simulink library "lib_component"  (Simulink 7.7)
settings: Solver=ode45  StartTime=0.0  StopTime=10.0  RelTol=1e-3
undefined symbols (not defined in the file): Earth, four_skew_D0, four_skew_D1, four_skew_D2, four_skew_D3, four_skew_D4, GAS_k, GAS_seed1, GAS_tau, GAS_Vnoise, GAS_Vref, GPS_position_noise, GPS_position_seed, GPS_time_noise, GPS_time_seed, GYRO_bx, GYRO_by, GYRO_bz, GYRO_nu, GYRO_nv, GYRO_omega, GYRO_seed1, GYRO_seed2, GYRO_zeta, MTQ_k, MTQ_tau, noise_sampling_rate, NSAS_ang_limit, NSAS_seed1, NSAS_seed2, NSAS_x_noise, NSAS_y_noise, RW_Gamp, RW_J, RW_kE, RW_kL, RW_kT, RW_LM, RW_RM, RW_Rsc, RW_T1, RW_T2, STT_AD_prob, STT_FOV, STT_moon_ang_limit, STT_sun_ang_limit, STT_x_noise, STT_y_noise, STT_z_noise, three_one_skew_D0, three_one_skew_D1, three_one_skew_D2, three_one_skew_D3, three_one_skew_D4, three_one_skew_matrix, WGS84
libraries: lib_component x11, simulink x5, aerolibutil x4, lib_util x2, lib_env x2, aerolibtransform2 x1, vrlib x1
settings Model: Creator=kkamiya  LastModifiedBy=yamaurashusaku

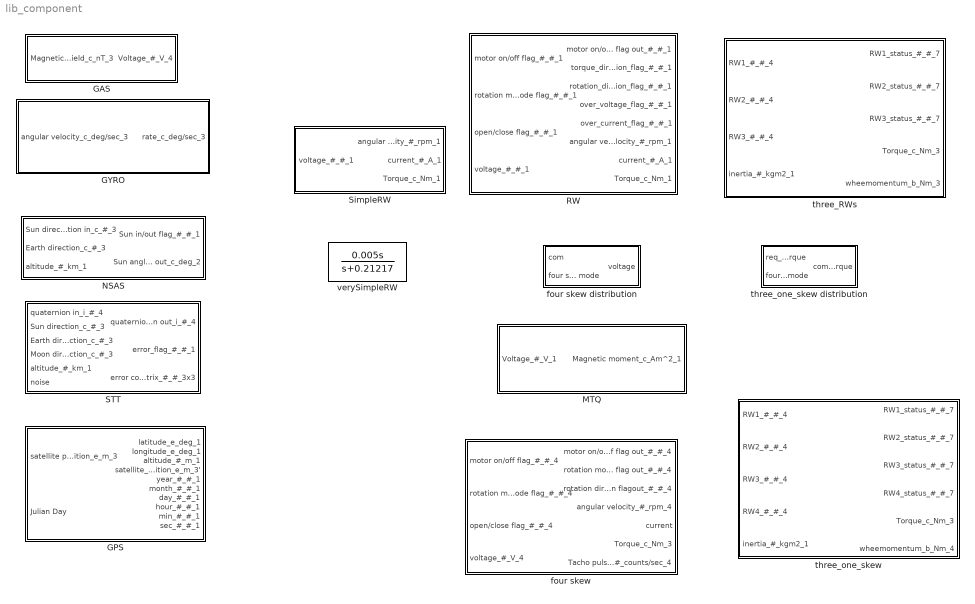
== system lib_component ==
  GAS : Subsystem
  GPS : Subsystem
  GYRO : Subsystem
  MTQ : Subsystem
  NSAS : Subsystem
  RW : Subsystem
  STT : Subsystem
  SimpleRW : Subsystem
  four skew : Subsystem
  four skew distribution : Subsystem
  three_RWs : Subsystem  AncestorBlock=lib_component/three_one_skew
  three_one_skew : Subsystem
  three_one_skew distribution : Subsystem
  verySimpleRW : TransferFcn  Numerator=[0.005 0]  Denominator=[1 0.21217]

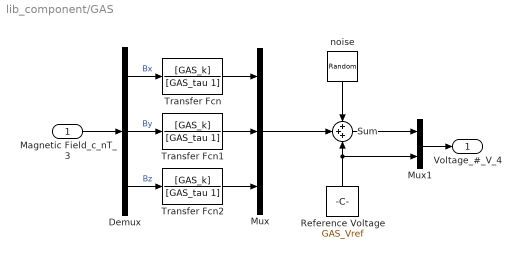
== system lib_component/GAS ==
  Magnetic Field_c_nT_3 : Inport
  Demux : Demux  Outputs=3
  Mux : Mux  Inputs=3
  Mux1 : Mux  Inputs=2
  Reference Voltage : Constant  Value=GAS_Vref
  Sum : Sum  Inputs=+++
  Transfer Fcn : TransferFcn  Numerator=[GAS_k]  Denominator=[GAS_tau 1]
  Transfer Fcn1 : TransferFcn  Numerator=[GAS_k]  Denominator=[GAS_tau 1]
  Transfer Fcn2 : TransferFcn  Numerator=[GAS_k]  Denominator=[GAS_tau 1]
  noise : RandomNumber  Mean=[0 0 0]  Variance=[GAS_Vnoise*GAS_Vnoise GAS_Vnoise*GAS_Vnoise GAS_Vnoise*GAS_Vnoise]  Seed=GAS_seed1  SampleTime=noise_sampling_rate
  Voltage_#_V_4 : Outport
  wires:
  Demux/2 -> Transfer Fcn1/1  "By"
  Demux/3 -> Transfer Fcn2/1  "Bz"
  Demux/1 -> Transfer Fcn/1  "Bx"
  Transfer Fcn2/1 -> Mux/3
  Transfer Fcn1/1 -> Mux/2
  Transfer Fcn/1 -> Mux/1
  Mux/1 -> Sum/2
  Mux1/1 -> Voltage_#_V_4/1
  Reference Voltage/1 -> Sum/3, Mux1/2
  Sum/1 -> Mux1/1
  Magnetic Field_c_nT_3/1 -> Demux/1
  noise/1 -> Sum/1

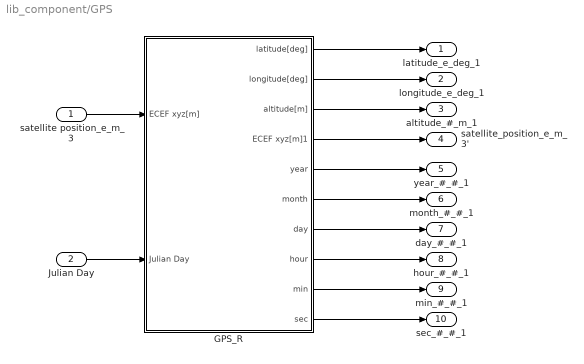
== system lib_component/GPS ==
  satellite position_e_m_3 : Inport
  Julian Day : Inport  Port=2
  GPS_R : Subsystem
  latitude_e_deg_1 : Outport
  longitude_e_deg_1 : Outport  Port=2
  altitude_#_m_1 : Outport  Port=3
  satellite_position_e_m_3' : Outport  Port=4
  year_#_#_1 : Outport  Port=5
  month_#_#_1 : Outport  Port=6
  day_#_#_1 : Outport  Port=7
  hour_#_#_1 : Outport  Port=8
  min_#_#_1 : Outport  Port=9
  sec_#_#_1 : Outport  Port=10
  wires:
  Julian Day/1 -> GPS_R/2(Julian Day)
  satellite position_e_m_3/1 -> GPS_R/1(ECEF xyz[m])
  GPS_R/1(latitude[deg]) -> latitude_e_deg_1/1
  GPS_R/2(longitude[deg]) -> longitude_e_deg_1/1
  GPS_R/3(altitude[m]) -> altitude_#_m_1/1
  GPS_R/4(ECEF xyz[m]1) -> satellite_position_e_m_3'/1
  GPS_R/5(year) -> year_#_#_1/1
  GPS_R/6(month) -> month_#_#_1/1
  GPS_R/7(day) -> day_#_#_1/1
  GPS_R/8(hour) -> hour_#_#_1/1
  GPS_R/9(min) -> min_#_#_1/1
  GPS_R/10(sec) -> sec_#_#_1/1

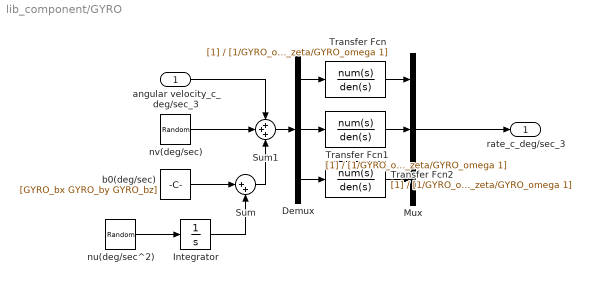
== system lib_component/GYRO ==
  angular velocity_c_deg/sec_3 : Inport
  Demux : Demux  Outputs=3
  Integrator : Integrator
  Mux : Mux  Inputs=3
  Sum : Sum  Inputs=|++
  Sum1 : Sum  Inputs=+++
  Transfer Fcn : TransferFcn  Denominator=[1/GYRO_omega/GYRO_omega 2*GYRO_zeta/GYRO_omega 1]
  Transfer Fcn1 : TransferFcn  Denominator=[1/GYRO_omega/GYRO_omega 2*GYRO_zeta/GYRO_omega 1]
  Transfer Fcn2 : TransferFcn  Denominator=[1/GYRO_omega/GYRO_omega 2*GYRO_zeta/GYRO_omega 1]
  b0(deg/sec) : Constant  Value=[GYRO_bx GYRO_by GYRO_bz]
  nu(deg/sec^2) : RandomNumber  Mean=[0 0 0]  Variance=[GYRO_nu*GYRO_nu GYRO_nu*GYRO_nu GYRO_nu*GYRO_nu]  Seed=GYRO_seed2  SampleTime=noise_sampling_rate
  nv(deg/sec) : RandomNumber  Mean=[0 0 0]  Variance=[GYRO_nv*GYRO_nv GYRO_nv*GYRO_nv GYRO_nv*GYRO_nv]  Seed=GYRO_seed1  SampleTime=noise_sampling_rate
  rate_c_deg/sec_3 : Outport
  wires:
  Transfer Fcn/1 -> Mux/1
  Transfer Fcn1/1 -> Mux/2
  Transfer Fcn2/1 -> Mux/3
  nu(deg/sec^2)/1 -> Integrator/1
  b0(deg/sec)/1 -> Sum/1
  nv(deg/sec)/1 -> Sum1/2
  Sum/1 -> Sum1/3
  angular velocity_c_deg/sec_3/1 -> Sum1/1
  Sum1/1 -> Demux/1
  Demux/2 -> Transfer Fcn1/1
  Demux/1 -> Transfer Fcn/1
  Demux/3 -> Transfer Fcn2/1
  Mux/1 -> rate_c_deg/sec_3/1
  Integrator/1 -> Sum/2

== system lib_component/MTQ ==
  Voltage_#_V_1 : Inport
  Transfer Fcn : TransferFcn  Numerator=[MTQ_k]  Denominator=[MTQ_tau 1]
  Magnetic moment_c_Am^2_1 : Outport
  wires:
  Voltage_#_V_1/1 -> Transfer Fcn/1
  Transfer Fcn/1 -> Magnetic moment_c_Am^2_1/1

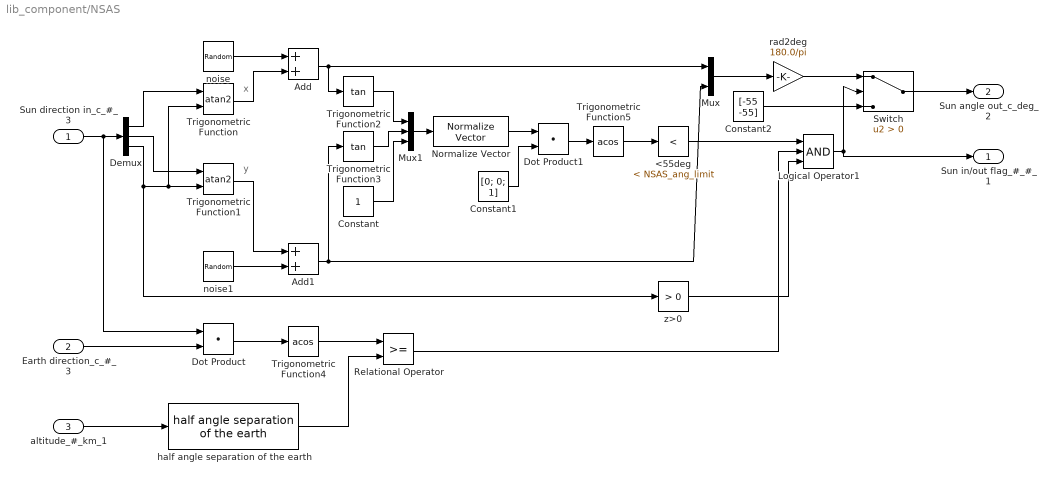
== system lib_component/NSAS ==
  note: x
  note: y
  Sun direction in_c_#_3 : Inport
  Earth direction_c_#_3 : Inport  Port=2
  altitude_#_km_1 : Inport  Port=3
  <55deg : simulink/Logic and Bit Operations/Compare To Constant  SystemSampleTime=-1  relop=<  const=NSAS_ang_limit  LogicOutDataTypeMode=uint8
  Add : Sum
  Add1 : Sum
  Constant : Constant
  Constant1 : Constant  Value=[0; 0; 1]
  Constant2 : Constant  Value=[-55 -55]
  Demux : Demux  Outputs=3
  Dot Product : DotProduct  InputSameDT=on  OutDataTypeStr=Inherit: Inherit via internal rule
  Dot Product1 : DotProduct  InputSameDT=on  OutDataTypeStr=Inherit: Inherit via internal rule
  Logical Operator1 : Logic  Inputs=3  AllPortsSameDT=off  OutDataTypeStr=boolean
  Mux : Mux  Inputs=2
  Mux1 : Mux  Inputs=3
  Normalize Vector : vrlib/Utilities/Normalize Vector  SystemSampleTime=-1  maxzero=0
  Relational Operator : RelationalOperator  OutDataTypeStr=boolean
  Switch : Switch  Criteria=u2 > Threshold
  Trigonometric Function : Trigonometry  Operator=atan2
  Trigonometric Function1 : Trigonometry  Operator=atan2
  Trigonometric Function2 : Trigonometry  Operator=tan
  Trigonometric Function3 : Trigonometry  Operator=tan
  Trigonometric Function4 : Trigonometry  Operator=acos
  Trigonometric Function5 : Trigonometry  Operator=acos
  half angle separation of the earth : lib_env/half angle separation of the earth  SystemSampleTime=-1
  noise : RandomNumber  Variance=NSAS_x_noise*NSAS_x_noise  Seed=NSAS_seed1  SampleTime=noise_sampling_rate
  noise1 : RandomNumber  Variance=NSAS_y_noise*NSAS_y_noise  Seed=NSAS_seed2  SampleTime=noise_sampling_rate
  rad2deg : Gain  Gain=180.0/pi
  z>0 : simulink/Logic and Bit Operations/Compare To Constant  SystemSampleTime=-1  relop=>  const=0  LogicOutDataTypeMode=uint8
  Sun in/out flag_#_#_1 : Outport
  Sun angle out_c_deg_2 : Outport  Port=2
  wires:
  noise1/1 -> Add1/2
  noise/1 -> Add/1
  Add/1 -> Mux/1, Trigonometric Function2/1
  Mux/1 -> rad2deg/1
  Switch/1 -> Sun angle out_c_deg_2/1
  Constant2/1 -> Switch/3
  Sun direction in_c_#_3/1 -> Demux/1, Dot Product/1
  Demux/2 -> Trigonometric Function1/1
  Demux/3 -> Trigonometric Function/2, Trigonometric Function1/2, z>0/1
  Demux/1 -> Trigonometric Function/1
  Trigonometric Function1/1 -> Add1/1
  Trigonometric Function/1 -> Add/2
  altitude_#_km_1/1 -> half angle separation of the earth/1
  Earth direction_c_#_3/1 -> Dot Product/2
  Dot Product/1 -> Trigonometric Function4/1
  half angle separation of the earth/1 -> Relational Operator/2
  Trigonometric Function4/1 -> Relational Operator/1
  Relational Operator/1 -> Logical Operator1/2
  Logical Operator1/1 -> Sun in/out flag_#_#_1/1, Switch/2
  Add1/1 -> Mux/2, Trigonometric Function3/1
  rad2deg/1 -> Switch/1
  <55deg/1 -> Logical Operator1/1
  Trigonometric Function2/1 -> Mux1/1
  Trigonometric Function3/1 -> Mux1/2
  Constant/1 -> Mux1/3
  Mux1/1 -> Normalize Vector/1
  Normalize Vector/1 -> Dot Product1/1
  Constant1/1 -> Dot Product1/2
  Dot Product1/1 -> Trigonometric Function5/1
  Trigonometric Function5/1 -> <55deg/1
  z>0/1 -> Logical Operator1/3

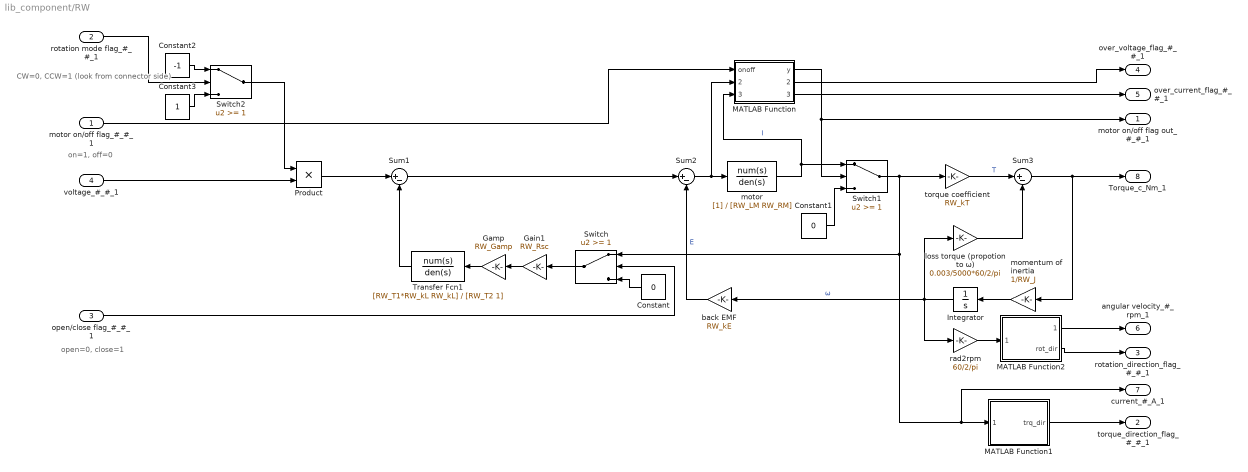
== system lib_component/RW ==
  note: CW=0, CCW=1
      | (look from connector side)
  note: open=0, close=1
  note: on=1, off=0
  motor on/off flag_#_#_1 : Inport
  rotation mode flag_#_#_1 : Inport  Port=2
  open/close flag_#_#_1 : Inport  Port=3
  voltage_#_#_1 : Inport  Port=4
  Constant : Constant  Value=0
  Constant1 : Constant  Value=0
  Constant2 : Constant  Value=-1
  Constant3 : Constant
  Gain1 : Gain  Gain=RW_Rsc
  Gamp : Gain  Gain=RW_Gamp
  Integrator : Integrator
  MATLAB Function : Stateflow chart  TreatAsAtomicUnit=on
  MATLAB Function1 : Stateflow chart  TreatAsAtomicUnit=on
  MATLAB Function2 : Stateflow chart  TreatAsAtomicUnit=on
  Product : Product  RndMeth=Zero
  Sum1 : Sum  Inputs=|+-
  Sum2 : Sum  Inputs=|+-
  Sum3 : Sum  Inputs=|+-
  Switch : Switch  Threshold=1
  Switch1 : Switch  Threshold=1
  Switch2 : Switch  Threshold=1
  Transfer Fcn1 : TransferFcn  Numerator=[RW_T1*RW_kL RW_kL]  Denominator=[RW_T2 1]
  back EMF : Gain  Gain=RW_kE
  loss torque (propotion to ω) : Gain  Gain=0.003/5000*60/2/pi
  momentum of inertia : Gain  Gain=1/RW_J
  motor : TransferFcn  Denominator=[RW_LM RW_RM]
  rad2rpm : Gain  Gain=60/2/pi
  torque coefficient : Gain  Gain=RW_kT
  motor on/off flag out_#_#_1 : Outport
  torque_direction_flag_#_#_1 : Outport  Port=2
  rotation_direction_flag_#_#_1 : Outport  Port=3
  over_voltage_flag_#_#_1 : Outport  Port=4
  over_current_flag_#_#_1 : Outport  Port=5
  angular velocity_#_rpm_1 : Outport  Port=6
  current_#_A_1 : Outport  Port=7
  Torque_c_Nm_1 : Outport  Port=8
  wires:
  Integrator/1 -> loss torque (propotion to ω)/1, back EMF/1, rad2rpm/1  "ω"
  momentum of inertia/1 -> Integrator/1
  torque coefficient/1 -> Sum3/1  "T"
  Sum2/1 -> motor/1, MATLAB Function/2(voltage)
  Gamp/1 -> Transfer Fcn1/1
  Gain1/1 -> Gamp/1
  rotation mode flag_#_#_1/1 -> Switch2/2
  open/close flag_#_#_1/1 -> Switch/2
  Constant/1 -> Switch/3
  Transfer Fcn1/1 -> Sum1/2
  Switch/1 -> Gain1/1
  rad2rpm/1 -> MATLAB Function2/1(omega)
  back EMF/1 -> Sum2/2  "E"
  Sum3/1 -> momentum of inertia/1, Torque_c_Nm_1/1
  loss torque (propotion to ω)/1 -> Sum3/2
  Constant2/1 -> Switch2/1
  Constant3/1 -> Switch2/3
  voltage_#_#_1/1 -> Product/2
  Switch2/1 -> Product/1
  Product/1 -> Sum1/1
  Switch1/1 -> torque coefficient/1, Switch/1, MATLAB Function1/1(current), current_#_A_1/1
  motor on/off flag_#_#_1/1 -> MATLAB Function/1(onoff)
  motor/1 -> Switch1/1, MATLAB Function/3(current)  "I"
  Constant1/1 -> Switch1/3
  MATLAB Function/1(y) -> Switch1/2, motor on/off flag out_#_#_1/1
  Sum1/1 -> Sum2/1
  MATLAB Function1/1(trq_dir) -> torque_direction_flag_#_#_1/1
  MATLAB Function2/2(rot_dir) -> rotation_direction_flag_#_#_1/1
  MATLAB Function2/1(omega_out) -> angular velocity_#_rpm_1/1
  MATLAB Function/2(over_voltage) -> over_voltage_flag_#_#_1/1
  MATLAB Function/3(over_current) -> over_current_flag_#_#_1/1

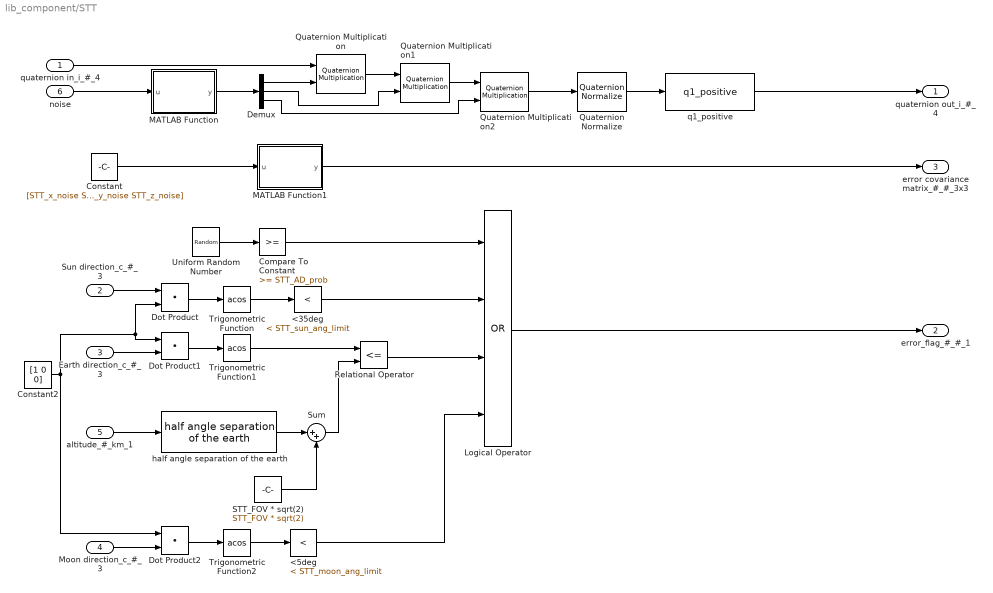
== system lib_component/STT ==
  quaternion in_i_#_4 : Inport
  Sun direction_c_#_3 : Inport  Port=2
  Earth direction_c_#_3 : Inport  Port=3
  Moon direction_c_#_3 : Inport  Port=4
  altitude_#_km_1 : Inport  Port=5
  noise : Inport  Port=6
  <35deg : simulink/Logic and Bit Operations/Compare To Constant  SystemSampleTime=-1  relop=<  const=STT_sun_ang_limit  LogicOutDataTypeMode=uint8
  <5deg : simulink/Logic and Bit Operations/Compare To Constant  SystemSampleTime=-1  relop=<  const=STT_moon_ang_limit  LogicOutDataTypeMode=uint8
  Compare To Constant : simulink/Logic and Bit Operations/Compare To Constant  SystemSampleTime=-1  relop=>=  const=STT_AD_prob  LogicOutDataTypeMode=uint8
  Constant : Constant  Value=[STT_x_noise STT_y_noise STT_z_noise]  SampleTime=0
  Constant2 : Constant  Value=[1 0 0]
  Demux : Demux  Outputs=3
  Dot Product : DotProduct  InputSameDT=on  OutDataTypeStr=Inherit: Inherit via internal rule
  Dot Product1 : DotProduct  InputSameDT=on  OutDataTypeStr=Inherit: Inherit via internal rule
  Dot Product2 : DotProduct  InputSameDT=on  OutDataTypeStr=Inherit: Inherit via internal rule
  Logical Operator : Logic  Operator=OR  Inputs=4  AllPortsSameDT=off  OutDataTypeStr=boolean
  MATLAB Function : Stateflow chart  TreatAsAtomicUnit=on
  MATLAB Function1 : Stateflow chart  TreatAsAtomicUnit=on
  Quaternion Multiplication : aerolibutil/Quaternion Multiplication  SystemSampleTime=-1
  Quaternion Multiplication1 : aerolibutil/Quaternion Multiplication  SystemSampleTime=-1
  Quaternion Multiplication2 : aerolibutil/Quaternion Multiplication  SystemSampleTime=-1
  Quaternion Normalize : aerolibutil/Quaternion Normalize  SystemSampleTime=-1
  Relational Operator : RelationalOperator  Operator=<=  OutDataTypeStr=boolean
  STT_FOV * sqrt(2) : Constant  Value=STT_FOV * sqrt(2)
  Sum : Sum  Inputs=|++
  Trigonometric Function : Trigonometry  Operator=acos
  Trigonometric Function1 : Trigonometry  Operator=acos
  Trigonometric Function2 : Trigonometry  Operator=acos
  Uniform Random Number : UniformRandomNumber  Minimum=0  SampleTime=noise_sampling_rate
  half angle separation of the earth : lib_env/half angle separation of the earth  SystemSampleTime=-1
  q1_positive : lib_util/q1_positive  SystemSampleTime=-1
  quaternion out_i_#_4 : Outport
  error_flag_#_#_1 : Outport  Port=2
  error covariance matrix_#_#_3x3 : Outport  Port=3
  wires:
  Dot Product2/1 -> Trigonometric Function2/1
  <5deg/1 -> Logical Operator/4
  Trigonometric Function2/1 -> <5deg/1
  Moon direction_c_#_3/1 -> Dot Product2/2
  <35deg/1 -> Logical Operator/2
  Trigonometric Function/1 -> <35deg/1
  Dot Product1/1 -> Trigonometric Function1/1
  Dot Product/1 -> Trigonometric Function/1
  Constant2/1 -> Dot Product2/1, Dot Product1/1, Dot Product/2
  Logical Operator/1 -> error_flag_#_#_1/1
  Compare To Constant/1 -> Logical Operator/1
  Earth direction_c_#_3/1 -> Dot Product1/2
  Sun direction_c_#_3/1 -> Dot Product/1
  Uniform Random Number/1 -> Compare To Constant/1
  quaternion in_i_#_4/1 -> Quaternion Multiplication/1
  MATLAB Function/1(y) -> Demux/1
  Demux/1 -> Quaternion Multiplication/2
  Quaternion Multiplication/1 -> Quaternion Multiplication1/1
  Demux/2 -> Quaternion Multiplication1/2
  Quaternion Multiplication1/1 -> Quaternion Multiplication2/1
  Demux/3 -> Quaternion Multiplication2/2
  Quaternion Multiplication2/1 -> Quaternion Normalize/1
  altitude_#_km_1/1 -> half angle separation of the earth/1
  half angle separation of the earth/1 -> Sum/1
  STT_FOV * sqrt(2)/1 -> Sum/2
  Relational Operator/1 -> Logical Operator/3
  Trigonometric Function1/1 -> Relational Operator/1
  Sum/1 -> Relational Operator/2
  MATLAB Function1/1(y) -> error covariance matrix_#_#_3x3/1
  Quaternion Normalize/1 -> q1_positive/1
  q1_positive/1 -> quaternion out_i_#_4/1
  Constant/1 -> MATLAB Function1/1(u)
  noise/1 -> MATLAB Function/1(u)

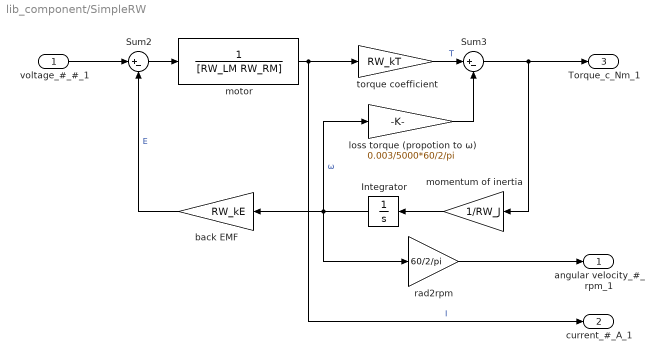
== system lib_component/SimpleRW ==
  voltage_#_#_1 : Inport
  Integrator : Integrator
  Sum2 : Sum  Inputs=|+-
  Sum3 : Sum  Inputs=|+-
  back EMF : Gain  Gain=RW_kE
  loss torque (propotion to ω) : Gain  Gain=0.003/5000*60/2/pi
  momentum of inertia : Gain  Gain=1/RW_J
  motor : TransferFcn  Denominator=[RW_LM RW_RM]
  rad2rpm : Gain  Gain=60/2/pi
  torque coefficient : Gain  Gain=RW_kT
  angular velocity_#_rpm_1 : Outport
  current_#_A_1 : Outport  Port=2
  Torque_c_Nm_1 : Outport  Port=3
  wires:
  motor/1 -> torque coefficient/1, current_#_A_1/1  "I"
  voltage_#_#_1/1 -> Sum2/1
  loss torque (propotion to ω)/1 -> Sum3/2
  Sum3/1 -> Torque_c_Nm_1/1, momentum of inertia/1
  back EMF/1 -> Sum2/2  "E"
  rad2rpm/1 -> angular velocity_#_rpm_1/1
  Sum2/1 -> motor/1
  torque coefficient/1 -> Sum3/1  "T"
  momentum of inertia/1 -> Integrator/1
  Integrator/1 -> rad2rpm/1, back EMF/1, loss torque (propotion to ω)/1  "ω"

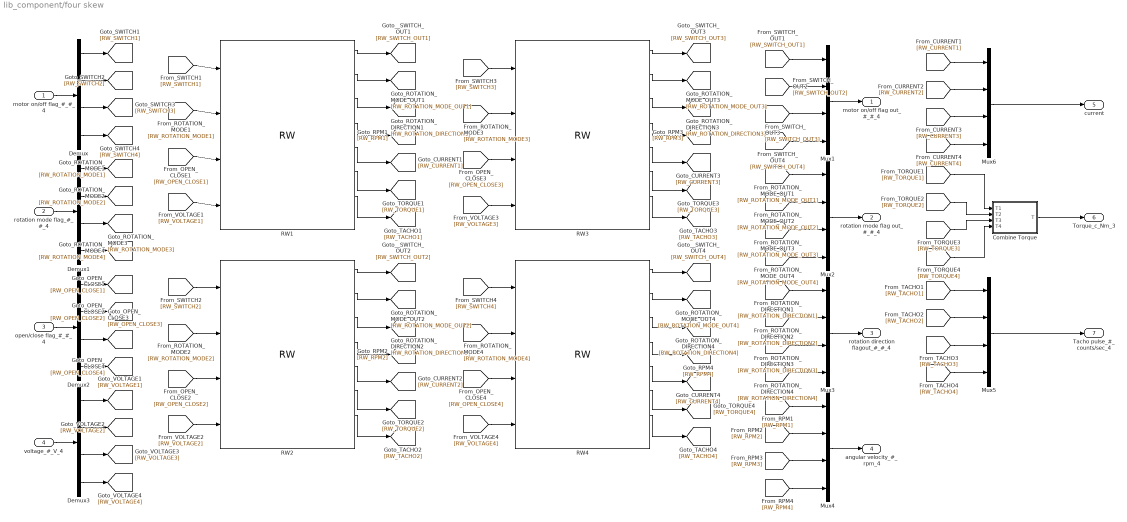
== system lib_component/four skew ==
  motor on/off flag_#_#_4 : Inport
  rotation mode flag_#_#_4 : Inport  Port=2
  open/close flag_#_#_4 : Inport  Port=3
  voltage_#_V_4 : Inport  Port=4
  Combine Torque : Stateflow chart  TreatAsAtomicUnit=on
  Demux{,1..3} (4 alike) : Demux
  Mux{1..6} (6 alike) : Mux
  RW{1..4} (4 alike) : lib_component/RW  SystemSampleTime=-1
  motor on/off flag out_#_#_4 : Outport
  rotation mode flag out_#_#_4 : Outport  Port=2
  rotation direction flagout_#_#_4 : Outport  Port=3
  angular velocity_#_rpm_4 : Outport  Port=4
  current : Outport  Port=5
  Torque_c_Nm_3 : Outport  Port=6
  Tacho pulse_#_counts/sec_4 : Outport  Port=7
  wires:
  Mux1/1 -> motor on/off flag out_#_#_4/1
  motor on/off flag_#_#_4/1 -> Demux/1
  Demux/1 -> [RW_SWITCH1]
  Demux/2 -> [RW_SWITCH2]
  Demux/3 -> [RW_SWITCH3]
  Demux/4 -> [RW_SWITCH4]
  [RW_SWITCH1] -> RW1/1
  [RW_ROTATION_MODE1] -> RW1/2
  [RW_OPEN_CLOSE1] -> RW1/3
  [RW_VOLTAGE1] -> RW1/4
  RW1/1 -> [RW_SWITCH_OUT1]
  RW1/2 -> [RW_ROTATION_MODE_OUT1]
  RW1/3 -> [RW_ROTATION_DIRECTION1]
  RW1/4 -> [RW_RPM1]
  RW1/5 -> [RW_CURRENT1]
  RW1/6 -> [RW_TORQUE1]
  RW1/7 -> [RW_TACHO1]
  [RW_SWITCH2] -> RW2/1
  [RW_ROTATION_MODE2] -> RW2/2
  [RW_OPEN_CLOSE2] -> RW2/3
  [RW_VOLTAGE2] -> RW2/4
  RW2/1 -> [RW_SWITCH_OUT2]
  RW2/2 -> [RW_ROTATION_MODE_OUT2]
  RW2/3 -> [RW_ROTATION_DIRECTION2]
  RW2/4 -> [RW_RPM2]
  RW2/5 -> [RW_CURRENT2]
  RW2/6 -> [RW_TORQUE2]
  RW2/7 -> [RW_TACHO2]
  Demux1/1 -> [RW_ROTATION_MODE1]
  Demux1/2 -> [RW_ROTATION_MODE2]
  Demux1/3 -> [RW_ROTATION_MODE3]
  Demux1/4 -> [RW_ROTATION_MODE4]
  rotation mode flag_#_#_4/1 -> Demux1/1
  Demux2/1 -> [RW_OPEN_CLOSE1]
  Demux2/2 -> [RW_OPEN_CLOSE2]
  Demux2/3 -> [RW_OPEN_CLOSE3]
  Demux2/4 -> [RW_OPEN_CLOSE4]
  open/close flag_#_#_4/1 -> Demux2/1
  Demux3/4 -> [RW_VOLTAGE4]
  Demux3/3 -> [RW_VOLTAGE3]
  Demux3/2 -> [RW_VOLTAGE2]
  Demux3/1 -> [RW_VOLTAGE1]
  voltage_#_V_4/1 -> Demux3/1
  [RW_SWITCH_OUT1] -> Mux1/1
  Mux2/1 -> rotation mode flag out_#_#_4/1
  Mux3/1 -> rotation direction flagout_#_#_4/1
  Mux4/1 -> angular velocity_#_rpm_4/1
  [RW_ROTATION_MODE_OUT1] -> Mux2/1
  [RW_SWITCH3] -> RW3/1
  [RW_ROTATION_MODE3] -> RW3/2
  [RW_OPEN_CLOSE3] -> RW3/3
  [RW_VOLTAGE3] -> RW3/4
  RW3/1 -> [RW_SWITCH_OUT3]
  RW3/2 -> [RW_ROTATION_MODE_OUT3]
  RW3/3 -> [RW_ROTATION_DIRECTION3]
  RW3/4 -> [RW_RPM3]
  RW3/5 -> [RW_CURRENT3]
  RW3/6 -> [RW_TORQUE3]
  RW3/7 -> [RW_TACHO3]
  [RW_SWITCH4] -> RW4/1
  [RW_ROTATION_MODE4] -> RW4/2
  [RW_OPEN_CLOSE4] -> RW4/3
  [RW_VOLTAGE4] -> RW4/4
  RW4/1 -> [RW_SWITCH_OUT4]
  RW4/2 -> [RW_ROTATION_MODE_OUT4]
  RW4/3 -> [RW_ROTATION_DIRECTION4]
  RW4/4 -> [RW_RPM4]
  RW4/5 -> [RW_CURRENT4]
  RW4/6 -> [RW_TORQUE4]
  RW4/7 -> [RW_TACHO4]
  Mux5/1 -> Tacho pulse_#_counts/sec_4/1
  Mux6/1 -> current/1
  [RW_ROTATION_DIRECTION1] -> Mux3/1
  [RW_RPM1] -> Mux4/1
  [RW_CURRENT1] -> Mux6/1
  [RW_TACHO1] -> Mux5/1
  [RW_TORQUE1] -> Combine Torque/1(T1)
  [RW_TORQUE2] -> Combine Torque/2(T2)
  [RW_TORQUE3] -> Combine Torque/3(T3)
  [RW_TORQUE4] -> Combine Torque/4(T4)
  [RW_SWITCH_OUT2] -> Mux1/2
  [RW_ROTATION_MODE_OUT2] -> Mux2/2
  [RW_ROTATION_DIRECTION2] -> Mux3/2
  [RW_RPM2] -> Mux4/2
  [RW_SWITCH_OUT3] -> Mux1/3
  [RW_ROTATION_MODE_OUT3] -> Mux2/3
  [RW_ROTATION_DIRECTION3] -> Mux3/3
  [RW_RPM3] -> Mux4/3
  [RW_SWITCH_OUT4] -> Mux1/4
  [RW_ROTATION_MODE_OUT4] -> Mux2/4
  [RW_ROTATION_DIRECTION4] -> Mux3/4
  [RW_RPM4] -> Mux4/4
  [RW_CURRENT2] -> Mux6/2
  [RW_TACHO2] -> Mux5/2
  [RW_CURRENT3] -> Mux6/3
  [RW_TACHO3] -> Mux5/3
  [RW_CURRENT4] -> Mux6/4
  [RW_TACHO4] -> Mux5/4
  Combine Torque/1(T) -> Torque_c_Nm_3/1

== system lib_component/four skew distribution ==
  com : Inport
  four skew mode : Inport  Port=2
  Multiport Switch : MultiPortSwitch  DataPortOrder=Specify indices  Inputs=5  DataPortIndices={0,1,2,3,4}  zeroidx=off
  Product : Product  Multiplication=Matrix(*)  RndMeth=Zero
  four_skew_D0 : Constant  Value=four_skew_D0
  four_skew_D1 : Constant  Value=four_skew_D1
  four_skew_D2 : Constant  Value=four_skew_D2
  four_skew_D3 : Constant  Value=four_skew_D3
  four_skew_D4 : Constant  Value=four_skew_D4
  voltage : Outport
  wires:
  Product/1 -> voltage/1
  Multiport Switch/1 -> Product/1
  com/1 -> Product/2
  four_skew_D4/1 -> Multiport Switch/6
  four_skew_D3/1 -> Multiport Switch/5
  four_skew_D2/1 -> Multiport Switch/4
  four_skew_D1/1 -> Multiport Switch/3
  four_skew_D0/1 -> Multiport Switch/2
  four skew mode/1 -> Multiport Switch/1

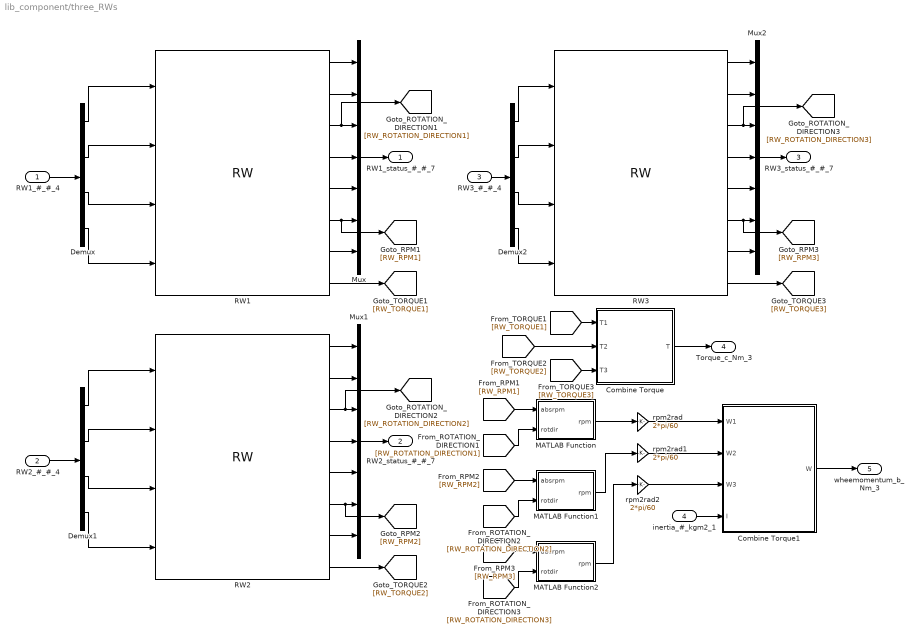
== system lib_component/three_RWs ==
  RW1_#_#_4 : Inport
  RW2_#_#_4 : Inport  Port=2
  RW3_#_#_4 : Inport  Port=3
  inertia_#_kgm2_1 : Inport  Port=4
  Combine Torque : Stateflow chart  TreatAsAtomicUnit=on
  Combine Torque1 : Stateflow chart  TreatAsAtomicUnit=on
  Demux : Demux
  Demux1 : Demux
  Demux2 : Demux
  MATLAB Function : Stateflow chart  TreatAsAtomicUnit=on
  MATLAB Function1 : Stateflow chart  TreatAsAtomicUnit=on
  MATLAB Function2 : Stateflow chart  TreatAsAtomicUnit=on
  Mux : Mux  Inputs=7
  Mux1 : Mux  Inputs=7
  Mux2 : Mux  Inputs=7
  RW1 : lib_component/RW  SystemSampleTime=-1
  RW2 : lib_component/RW  SystemSampleTime=-1
  RW3 : lib_component/RW  SystemSampleTime=-1
  rpm2rad : Gain  Gain=2*pi/60
  rpm2rad1 : Gain  Gain=2*pi/60
  rpm2rad2 : Gain  Gain=2*pi/60
  RW1_status_#_#_7 : Outport
  RW2_status_#_#_7 : Outport  Port=2
  RW3_status_#_#_7 : Outport  Port=3
  Torque_c_Nm_3 : Outport  Port=4
  wheemomentum_b_Nm_3 : Outport  Port=5
  wires:
  rpm2rad2/1 -> Combine Torque1/3(W3)
  rpm2rad1/1 -> Combine Torque1/2(W2)
  rpm2rad/1 -> Combine Torque1/1(W1)
  inertia_#_kgm2_1/1 -> Combine Torque1/4(I)
  Combine Torque1/1(W) -> wheemomentum_b_Nm_3/1
  RW1_#_#_4/1 -> Demux/1
  RW2_#_#_4/1 -> Demux1/1
  [RW_TORQUE1] -> Combine Torque/1(T1)
  [RW_TORQUE2] -> Combine Torque/2(T2)
  [RW_TORQUE3] -> Combine Torque/3(T3)
  Combine Torque/1(T) -> Torque_c_Nm_3/1
  Demux/1 -> RW1/1
  Demux/2 -> RW1/2
  Demux/3 -> RW1/3
  Demux/4 -> RW1/4
  RW3_#_#_4/1 -> Demux2/1
  Demux1/1 -> RW2/1
  Demux1/2 -> RW2/2
  Demux1/3 -> RW2/3
  Demux1/4 -> RW2/4
  Demux2/1 -> RW3/1
  Demux2/2 -> RW3/2
  Demux2/3 -> RW3/3
  Demux2/4 -> RW3/4
  RW1/1 -> Mux/1
  RW1/2 -> Mux/2
  RW1/3 -> Mux/3, [RW_ROTATION_DIRECTION1]
  RW1/4 -> Mux/4
  RW1/5 -> Mux/5
  RW1/6 -> Mux/6, [RW_RPM1]
  RW1/7 -> Mux/7
  RW1/8 -> [RW_TORQUE1]
  Mux/1 -> RW1_status_#_#_7/1
  [RW_RPM1] -> MATLAB Function/1(absrpm)
  [RW_ROTATION_DIRECTION1] -> MATLAB Function/2(rotdir)
  [RW_RPM2] -> MATLAB Function1/1(absrpm)
  [RW_ROTATION_DIRECTION2] -> MATLAB Function1/2(rotdir)
  [RW_RPM3] -> MATLAB Function2/1(absrpm)
  [RW_ROTATION_DIRECTION3] -> MATLAB Function2/2(rotdir)
  MATLAB Function2/1(rpm) -> rpm2rad2/1
  MATLAB Function1/1(rpm) -> rpm2rad1/1
  MATLAB Function/1(rpm) -> rpm2rad/1
  RW2/1 -> Mux1/1
  RW2/2 -> Mux1/2
  RW2/3 -> Mux1/3, [RW_ROTATION_DIRECTION2]
  RW2/4 -> Mux1/4
  RW2/5 -> Mux1/5
  RW2/6 -> Mux1/6, [RW_RPM2]
  RW2/7 -> Mux1/7
  RW2/8 -> [RW_TORQUE2]
  Mux1/1 -> RW2_status_#_#_7/1
  RW3/1 -> Mux2/1
  RW3/2 -> Mux2/2
  RW3/3 -> Mux2/3, [RW_ROTATION_DIRECTION3]
  RW3/4 -> Mux2/4
  RW3/5 -> Mux2/5
  RW3/6 -> Mux2/6, [RW_RPM3]
  RW3/7 -> Mux2/7
  RW3/8 -> [RW_TORQUE3]
  Mux2/1 -> RW3_status_#_#_7/1

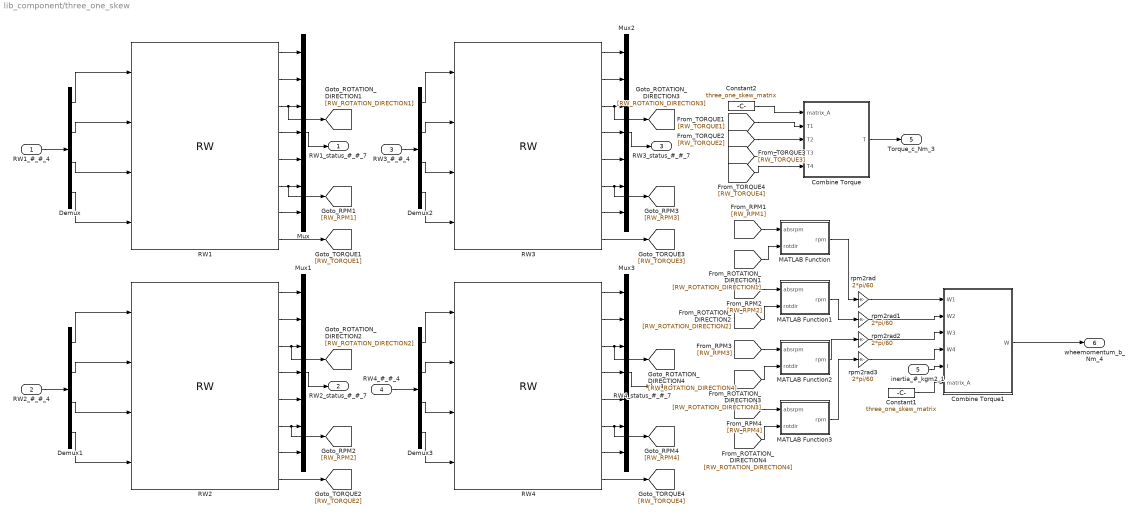
== system lib_component/three_one_skew ==
  RW1_#_#_4 : Inport
  RW2_#_#_4 : Inport  Port=2
  RW3_#_#_4 : Inport  Port=3
  RW4_#_#_4 : Inport  Port=4
  inertia_#_kgm2_1 : Inport  Port=5
  Combine Torque : Stateflow chart  TreatAsAtomicUnit=on
  Combine Torque1 : Stateflow chart  TreatAsAtomicUnit=on
  Constant1 : Constant  Value=three_one_skew_matrix
  Constant2 : Constant  Value=three_one_skew_matrix
  Demux{,1..3} (4 alike) : Demux
  MATLAB Function : Stateflow chart  TreatAsAtomicUnit=on
  MATLAB Function1 : Stateflow chart  TreatAsAtomicUnit=on
  MATLAB Function2 : Stateflow chart  TreatAsAtomicUnit=on
  MATLAB Function3 : Stateflow chart  TreatAsAtomicUnit=on
  Mux{,1..3} (4 alike) : Mux  Inputs=7
  RW{1..4} (4 alike) : lib_component/RW  SystemSampleTime=-1
  rpm2rad{,1..3} (4 alike) : Gain  Gain=2*pi/60
  RW1_status_#_#_7 : Outport
  RW2_status_#_#_7 : Outport  Port=2
  RW3_status_#_#_7 : Outport  Port=3
  RW4_status_#_#_7 : Outport  Port=4
  Torque_c_Nm_3 : Outport  Port=5
  wheemomentum_b_Nm_4 : Outport  Port=6
  wires:
  rpm2rad3/1 -> Combine Torque1/4(W4)
  rpm2rad2/1 -> Combine Torque1/3(W3)
  rpm2rad1/1 -> Combine Torque1/2(W2)
  rpm2rad/1 -> Combine Torque1/1(W1)
  inertia_#_kgm2_1/1 -> Combine Torque1/5(I)
  Combine Torque1/1(W) -> wheemomentum_b_Nm_4/1
  RW1_#_#_4/1 -> Demux/1
  RW2_#_#_4/1 -> Demux1/1
  RW4_#_#_4/1 -> Demux3/1
  [RW_TORQUE1] -> Combine Torque/2(T1)
  [RW_TORQUE2] -> Combine Torque/3(T2)
  [RW_TORQUE3] -> Combine Torque/4(T3)
  [RW_TORQUE4] -> Combine Torque/5(T4)
  Combine Torque/1(T) -> Torque_c_Nm_3/1
  Constant2/1 -> Combine Torque/1(matrix_A)
  Constant1/1 -> Combine Torque1/6(matrix_A)
  Demux/1 -> RW1/1
  Demux/2 -> RW1/2
  Demux/3 -> RW1/3
  Demux/4 -> RW1/4
  RW3_#_#_4/1 -> Demux2/1
  Demux1/1 -> RW2/1
  Demux1/2 -> RW2/2
  Demux1/3 -> RW2/3
  Demux1/4 -> RW2/4
  Demux2/1 -> RW3/1
  Demux2/2 -> RW3/2
  Demux2/3 -> RW3/3
  Demux2/4 -> RW3/4
  Demux3/1 -> RW4/1
  Demux3/2 -> RW4/2
  Demux3/3 -> RW4/3
  Demux3/4 -> RW4/4
  RW1/1 -> Mux/1
  RW1/2 -> Mux/2
  RW1/3 -> Mux/3, [RW_ROTATION_DIRECTION1]
  RW1/4 -> Mux/4
  RW1/5 -> Mux/5
  RW1/6 -> Mux/6, [RW_RPM1]
  RW1/7 -> Mux/7
  RW1/8 -> [RW_TORQUE1]
  Mux/1 -> RW1_status_#_#_7/1
  [RW_RPM1] -> MATLAB Function/1(absrpm)
  [RW_ROTATION_DIRECTION1] -> MATLAB Function/2(rotdir)
  [RW_RPM2] -> MATLAB Function1/1(absrpm)
  [RW_ROTATION_DIRECTION2] -> MATLAB Function1/2(rotdir)
  [RW_RPM3] -> MATLAB Function2/1(absrpm)
  [RW_ROTATION_DIRECTION3] -> MATLAB Function2/2(rotdir)
  [RW_RPM4] -> MATLAB Function3/1(absrpm)
  [RW_ROTATION_DIRECTION4] -> MATLAB Function3/2(rotdir)
  MATLAB Function3/1(rpm) -> rpm2rad3/1
  MATLAB Function2/1(rpm) -> rpm2rad2/1
  MATLAB Function1/1(rpm) -> rpm2rad1/1
  MATLAB Function/1(rpm) -> rpm2rad/1
  RW2/1 -> Mux1/1
  RW2/2 -> Mux1/2
  RW2/3 -> Mux1/3, [RW_ROTATION_DIRECTION2]
  RW2/4 -> Mux1/4
  RW2/5 -> Mux1/5
  RW2/6 -> Mux1/6, [RW_RPM2]
  RW2/7 -> Mux1/7
  RW2/8 -> [RW_TORQUE2]
  Mux1/1 -> RW2_status_#_#_7/1
  RW3/1 -> Mux2/1
  RW3/2 -> Mux2/2
  RW3/3 -> Mux2/3, [RW_ROTATION_DIRECTION3]
  RW3/4 -> Mux2/4
  RW3/5 -> Mux2/5
  RW3/6 -> Mux2/6, [RW_RPM3]
  RW3/7 -> Mux2/7
  RW3/8 -> [RW_TORQUE3]
  Mux2/1 -> RW3_status_#_#_7/1
  RW4/1 -> Mux3/1
  RW4/2 -> Mux3/2
  RW4/3 -> Mux3/3, [RW_ROTATION_DIRECTION4]
  RW4/4 -> Mux3/4
  RW4/5 -> Mux3/5
  RW4/6 -> Mux3/6, [RW_RPM4]
  RW4/7 -> Mux3/7
  RW4/8 -> [RW_TORQUE4]
  Mux3/1 -> RW4_status_#_#_7/1

== system lib_component/three_one_skew distribution ==
  req_torque : Inport
  four skew mode : Inport  Port=2
  Multiport Switch : MultiPortSwitch  DataPortOrder=Specify indices  Inputs=5  DataPortIndices={0,1,2,3,4}  zeroidx=off
  Product : Product  Multiplication=Matrix(*)  RndMeth=Zero
  three_one_skew_D0 : Constant  Value=three_one_skew_D0
  three_one_skew_D1 : Constant  Value=three_one_skew_D1
  three_one_skew_D2 : Constant  Value=three_one_skew_D2
  three_one_skew_D3 : Constant  Value=three_one_skew_D3
  three_one_skew_D4 : Constant  Value=three_one_skew_D4
  com_torque : Outport
  wires:
  Product/1 -> com_torque/1
  Multiport Switch/1 -> Product/1
  req_torque/1 -> Product/2
  three_one_skew_D4/1 -> Multiport Switch/6
  three_one_skew_D3/1 -> Multiport Switch/5
  three_one_skew_D2/1 -> Multiport Switch/4
  three_one_skew_D1/1 -> Multiport Switch/3
  three_one_skew_D0/1 -> Multiport Switch/2
  four skew mode/1 -> Multiport Switch/1

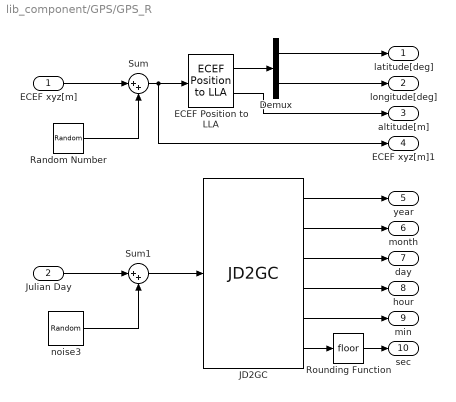
== system lib_component/GPS/GPS_R ==
  ECEF xyz[m] : Inport
  Julian Day : Inport  Port=2
  Demux : Demux  Outputs=2
  ECEF Position to LLA : aerolibtransform2/ECEF Position to LLA  SystemSampleTime=-1  units=Metric (MKS)  ptype=Earth (WGS84)  F=1/298.257223563  R=6378137
  JD2GC : lib_util/JD2GC  SystemSampleTime=-1
  Random Number : RandomNumber  Mean=[0 0 0]  Variance=[GPS_position_noise*GPS_position_noise GPS_position_noise*GPS_position_noise GPS_position_noise*GPS_position_noise]  Seed=GPS_position_seed  SampleTime=noise_sampling_rate
  Rounding Function : Rounding
  Sum : Sum  Inputs=|++
  Sum1 : Sum  Inputs=|++
  noise3 : UniformRandomNumber  Minimum=0  Maximum=GPS_time_noise  Seed=GPS_time_seed  SampleTime=noise_sampling_rate
  latitude[deg] : Outport
  longitude[deg] : Outport  Port=2
  altitude[m] : Outport  Port=3
  ECEF xyz[m]1 : Outport  Port=4
  year : Outport  Port=5
  month : Outport  Port=6
  day : Outport  Port=7
  hour : Outport  Port=8
  min : Outport  Port=9
  sec : Outport  Port=10
  wires:
  Sum1/1 -> JD2GC/1
  Julian Day/1 -> Sum1/1
  noise3/1 -> Sum1/2
  ECEF Position to LLA/2 -> altitude[m]/1
  Demux/1 -> latitude[deg]/1
  Demux/2 -> longitude[deg]/1
  ECEF Position to LLA/1 -> Demux/1
  Sum/1 -> ECEF xyz[m]1/1, ECEF Position to LLA/1
  Random Number/1 -> Sum/2
  JD2GC/6 -> Rounding Function/1
  JD2GC/5 -> min/1
  JD2GC/4 -> hour/1
  JD2GC/3 -> day/1
  JD2GC/2 -> month/1
  JD2GC/1 -> year/1
  ECEF xyz[m]/1 -> Sum/1
  Rounding Function/1 -> sec/1

== matlab function four skew/Combine Torque ==
  data: T1 input double; T output double; T2 input double; T3 input double; T4 input double
function T = four_skew_combine(T1, T2, T3, T4)
%#codegen

gamma = asin(1.0 / sqrt(3.0));

Tx = 1.0 / sqrt(2.0) * (T1 + T2 - T3 - T4) * cos(gamma);
Ty =                   (T1 + T2 + T3 + T4) * sin(gamma);
Tz = 1.0 / sqrt(2.0) * (T1 - T2 - T3 + T4) * cos(gamma);

T = [Tx; Ty; Tz];

== matlab function three_one_skew/Combine Torque ==
  data: matrix_A input double; T1 input double; T output double; T2 input double; T3 input double; T4 input double
function T = four_skew_combine(matrix_A,T1, T2, T3, T4)
%#codegen

% T=three_one_skew_matrix*[T1;T2;T3;T4];
T=matrix_A*[T1;T2;T3;T4];

== matlab function three_one_skew/Combine Torque1 ==
  data: W1 input double; W output double; W2 input double; W3 input double; W4 input double; I input double; matrix_A input double
function W = four_skew_combine(W1, W2, W3, W4, I,matrix_A)
%#codegen

% W=three_one_skew_matrix*I*[W1;W2;W3;W4];
W=matrix_A*I*[W1;W2;W3;W4];

== matlab function STT/MATLAB Function ==
  data: u input double; y output double
function y = fcn(u)
%#codegen

qx = [cos(u(1)/2.0) sin(u(1)/2.0) 0 0];
qy = [cos(u(2)/2.0) 0 sin(u(2)/2.0) 0];
qz = [cos(u(3)/2.0) 0 0 sin(u(3)/2.0)];

y = [qx qy qz];

== matlab function STT/MATLAB Function1 ==
  data: u input double; y output double
function y = fcn(u)
%#codegen

dx = sin(u(1)/2.0);
dy = sin(u(2)/2.0);
dz = sin(u(3)/2.0);

y = [dx * dx 0 0; 0 dy * dy 0; 0 0 dz * dz];

== matlab function RW/MATLAB Function ==
  data: onoff input double; y output double; voltage input double; current input double; over_voltage output double; over_current output double
function [y,over_voltage,over_current]= fcn(onoff,voltage,current)
%#codegen

y = 1;
over_voltage = 0;
over_current = 0;

if onoff == 0
    y = 0;
end

if abs(voltage) > 37
    y = 0;
    over_voltage = 1;
end

if abs(current) > 3
    y = 0;
    over_current = 1;
end

== matlab function RW/MATLAB Function1 ==
  data: current input double; trq_dir output double
function trq_dir= fcn(current)
%#codegen

if current > 0
    trq_dir = 0;
else
    trq_dir = 1;
end

== matlab function RW/MATLAB Function2 ==
  data: omega_out output double; omega input double; rot_dir output double
function [omega_out, rot_dir]= fcn(omega)
%#codegen

if omega > 0
    rot_dir = 0;
else
    rot_dir = 1;
end

omega_out = abs(omega);

== matlab function three_one_skew/MATLAB Function ==
  data: absrpm input double; rpm output double; rotdir input double
function rpm = fcn(absrpm,rotdir)
%#codegen

rpm = absrpm;

if rotdir == 1
    rpm = -1 * rpm;
end

== matlab function three_one_skew/MATLAB Function1 ==
  data: absrpm input double; rpm output double; rotdir input double
function rpm = fcn(absrpm,rotdir)
%#codegen

rpm = absrpm;

if rotdir == 1
    rpm = -1 * rpm;
end

== matlab function three_one_skew/MATLAB Function2 ==
  data: absrpm input double; rpm output double; rotdir input double
function rpm = fcn(absrpm,rotdir)
%#codegen

rpm = absrpm;

if rotdir == 1
    rpm = -1 * rpm;
end

== matlab function three_one_skew/MATLAB Function3 ==
  data: absrpm input double; rpm output double; rotdir input double
function rpm = fcn(absrpm,rotdir)
%#codegen

rpm = absrpm;

if rotdir == 1
    rpm = -1 * rpm;
end

== matlab function three_RWs/Combine Torque ==
  data: T1 input double; T output double; T2 input double; T3 input double
function T = four_skew_combine(T1, T2, T3)
%#codegen

% T=three_one_skew_matrix*[T1;T2;T3;T4];
T=[T1;T2;T3];

== matlab function three_RWs/Combine Torque1 ==
  data: W1 input double; W output double; W2 input double; W3 input double; I input double
function W = four_skew_combine(W1, W2, W3, I)
%#codegen

% W=three_one_skew_matrix*I*[W1;W2;W3;W4];
W=I*[W1;W2;W3];

== matlab function three_RWs/MATLAB Function ==
  data: absrpm input double; rpm output double; rotdir input double
function rpm = fcn(absrpm,rotdir)
%#codegen

rpm = absrpm;

if rotdir == 1
    rpm = -1 * rpm;
end

== matlab function three_RWs/MATLAB Function1 ==
  data: absrpm input double; rpm output double; rotdir input double
function rpm = fcn(absrpm,rotdir)
%#codegen

rpm = absrpm;

if rotdir == 1
    rpm = -1 * rpm;
end

== matlab function three_RWs/MATLAB Function2 ==
  data: absrpm input double; rpm output double; rotdir input double
function rpm = fcn(absrpm,rotdir)
%#codegen

rpm = absrpm;

if rotdir == 1
    rpm = -1 * rpm;
end
